simulink library "avlAerodynamics2D"  (R2018b)
settings: Solver=VariableStepAuto  StartTime=0.0  StopTime=10.0  RelTol=1e-3
values from neighbouring files (symbols this model uses):
  Bref = dsgnData.Bref    [avlAerodynamics2D_ts.m]
  Cref = dsgnData.Cref    [avlAerodynamics2D_ts.m]
  k_CS_gain = calculate_2D_gains(dsgnTest_1,nom_a,nom_b,df,da,de,dr)    [avlAero2DCoeffs_ts.m]
  rho_fluid = 1    [avlAerodynamics2D_ts.m]
  Sref = dsgnData.Sref    [avlAerodynamics2D_ts.m]
undefined symbols (not defined in the file or in its folder): CDtot_2D_Tbl, CLtot_2D_Tbl, Cltot_2D_Tbl, Cmtot_2D_Tbl, Cntot_2D_Tbl
libraries: eulAng2RotMat_ul x1, alphaBeta_ul x1, avlAero2DCoeffs_ul x1
settings Model: Creator=mcobb  LastModifiedBy=Ayaz

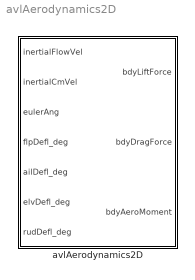
== system avlAerodynamics2D ==
  avlAerodynamics2D : Subsystem  mask{CLTable=CLtot_2D_Tbl, CDTable=CDtot_2D_Tbl, CMxTable=Cltot_2D_Tbl, CMyTable=Cmtot_2D_Tbl, CMzTable=Cntot_2D_Tbl, CsGainMatrix=k_CS_gain, SRef=Sref, BRef=Bref, CRef=Cref, rho_fluid=rho_fluid}
      mask prompts: CLTable "CL lookup table object"; CDTable "CD lookup table object"; CMxTable "CMx lookup table object"; CMyTable "CMy lookup table object"; CMzTable "CMz lookup table object"; CsGainMatrix "Control surface gain matrix"; SRef "Ref area (AVL Sref)"; BRef "Roll & Yaw Moment Reference Length (AVL Bref)"; CRef "Pitch Moment Reference Length (AVL Cref)"; rho_fluid "Fluid density"
      mask TypeOptions CLTable: avlAero2DCoeffs/CLTable
      mask TypeOptions CDTable: avlAero2DCoeffs/CDTable
      mask TypeOptions CMxTable: avlAero2DCoeffs/CMxTable
      mask TypeOptions CMyTable: avlAero2DCoeffs/CMyTable
      mask TypeOptions CMzTable: avlAero2DCoeffs/CMzTable
      mask TypeOptions CsGainMatrix: avlAero2DCoeffs/CsGainMatrix
      mask DialogControl Container4 Prompt: Reference Areas
      mask DialogControl Container5 Prompt: Environment

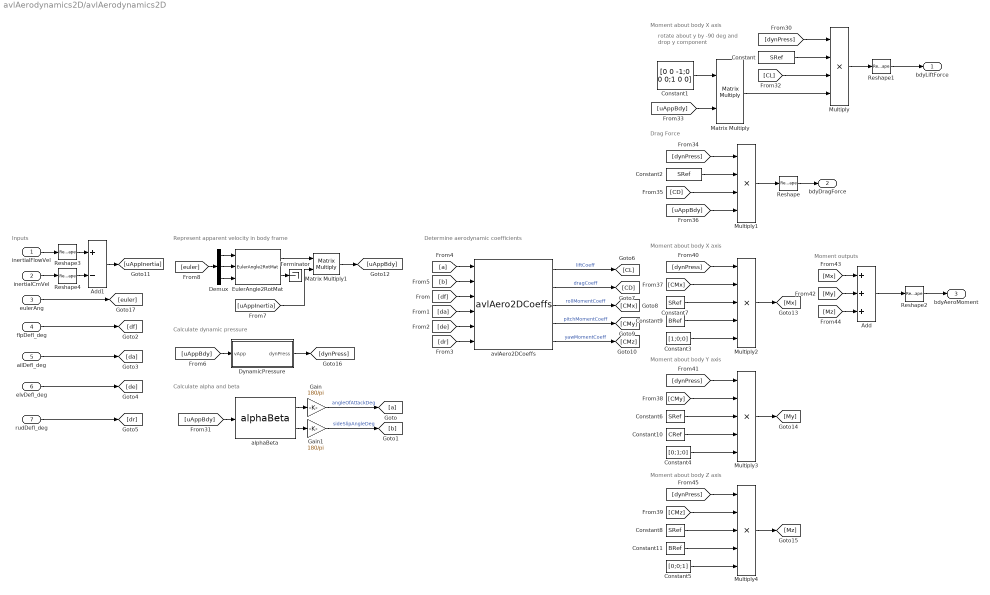
== system avlAerodynamics2D/avlAerodynamics2D ==
  note: Calculate dynamic pressure
  note: Represent apparent velocity in body frame
  note: Moment outputs
  note: Inputs
  note: Calculate alpha and beta
  note: Determine aerodynamic coefficients
  note: Moment about body X axis
  note: rotate about y by -90 deg
      | and drop y component
  note: Moment about body Y axis
  note: Moment about body Z axis
  note: Drag Force
  note: Moment about body X axis
  inertialFlowVel : Inport
  inertialCmVel : Inport  Port=2
  eulerAng : Inport  Port=3
  flpDefl_deg : Inport  Port=4
  ailDefl_deg : Inport  Port=5
  elvDefl_deg : Inport  Port=6
  rudDefl_deg : Inport  Port=7
  Add : Sum  Inputs=+++
  Add1 : Sum  Inputs=+-
  Constant{,2,6..8} (5 alike) : Constant  Value=SRef
  Constant1 : Constant  Value=[0 0 -1;0 0 0;1 0 0]
  Constant10 : Constant  Value=CRef
  Constant11 : Constant  Value=BRef
  Constant3 : Constant  Value=[1;0;0]  VectorParams1D=off
  Constant4 : Constant  Value=[0;1;0]  VectorParams1D=off
  Constant5 : Constant  Value=[0;0;1]  VectorParams1D=off
  Constant9 : Constant  Value=BRef
  Demux : Demux  Outputs=3
  DynamicPressure : Subsystem  mask{rho=rho_fluid}
      mask prompts: rho "Fluid density"
  EulerAngle2RotMat : eulAng2RotMat_ul/EulerAngle2RotMat  SystemSampleTime=-1
  Gain : Gain  Gain=180/pi
  Gain1 : Gain  Gain=180/pi
  Matrix Multiply : Product  Multiplication=Matrix(*)
  Matrix Multiply1 : Product  Multiplication=Matrix(*)
  Multiply : Product  Inputs=4
  Multiply1 : Product  Inputs=4
  Multiply2 : Product  Inputs=5
  Multiply3 : Product  Inputs=5
  Multiply4 : Product  Inputs=5
  Reshape{,1..4} (5 alike) : Reshape  OutputDimensionality=Column vector (2-D)
  Terminator : Terminator
  alphaBeta : alphaBeta_ul/alphaBeta  SystemSampleTime=-1
  avlAero2DCoeffs : avlAero2DCoeffs_ul/avlAero2DCoeffs  CLTable=CLTable  CDTable=CDTable  CMxTable=CMxTable  CMyTable=CMyTable  CMzTable=CMzTable  CsGainMatrix=CsGainMatrix
  bdyLiftForce : Outport
  bdyDragForce : Outport  Port=2
  bdyAeroMoment : Outport  Port=3
  wires:
  flpDefl_deg/1 -> [df]
  ailDefl_deg/1 -> [da]
  elvDefl_deg/1 -> [de]
  rudDefl_deg/1 -> [dr]
  alphaBeta/1 -> Gain/1
  alphaBeta/2 -> Gain1/1
  Gain/1 -> [a]  "angleOfAttackDeg"
  Gain1/1 -> [b]  "sideSlipAngleDeg"
  [uAppBdy] -> alphaBeta/1
  [dynPress] -> Multiply/1
  Constant/1 -> Multiply/2
  [CL] -> Multiply/3
  Matrix Multiply/1 -> Multiply/4
  Constant1/1 -> Matrix Multiply/1
  [uAppBdy] -> Matrix Multiply/2
  [CD] -> Multiply1/3
  Constant2/1 -> Multiply1/2
  [dynPress] -> Multiply1/1
  [uAppBdy] -> Multiply1/4
  Multiply/1 -> Reshape1/1
  Multiply1/1 -> Reshape/1
  Reshape1/1 -> bdyLiftForce/1
  Reshape/1 -> bdyDragForce/1
  [CMx] -> Multiply2/2
  Multiply2/1 -> [Mx]
  Multiply3/1 -> [My]
  [CMy] -> Multiply3/2
  [CMz] -> Multiply4/2
  Multiply4/1 -> [Mz]
  [My] -> Add/2
  [Mx] -> Add/1
  [Mz] -> Add/3
  Add/1 -> Reshape2/1
  Reshape2/1 -> bdyAeroMoment/1
  Reshape3/1 -> Add1/1
  Constant7/1 -> Multiply2/3
  Constant6/1 -> Multiply3/3
  Constant8/1 -> Multiply4/3
  Constant3/1 -> Multiply2/5
  Constant4/1 -> Multiply3/5
  Constant5/1 -> Multiply4/5
  [dynPress] -> Multiply3/1
  [dynPress] -> Multiply4/1
  Constant9/1 -> Multiply2/4
  [dynPress] -> Multiply2/1
  Constant10/1 -> Multiply3/4
  Constant11/1 -> Multiply4/4
  [dr] -> avlAero2DCoeffs/6
  [de] -> avlAero2DCoeffs/5
  [da] -> avlAero2DCoeffs/4
  [df] -> avlAero2DCoeffs/3
  avlAero2DCoeffs/5 -> [CMz]  "yawMomentCoeff"
  avlAero2DCoeffs/4 -> [CMy]  "pitchMomentCoeff"
  avlAero2DCoeffs/3 -> [CMx]  "rollMomentCoeff"
  avlAero2DCoeffs/2 -> [CD]  "dragCoeff"
  avlAero2DCoeffs/1 -> [CL]  "liftCoeff"
  Reshape4/1 -> Add1/2
  eulerAng/1 -> [euler]
  inertialCmVel/1 -> Reshape4/1
  inertialFlowVel/1 -> Reshape3/1
  Add1/1 -> [uAppInertia]
  Demux/1 -> EulerAngle2RotMat/1
  Demux/2 -> EulerAngle2RotMat/2
  Demux/3 -> EulerAngle2RotMat/3
  [euler] -> Demux/1
  EulerAngle2RotMat/2 -> Terminator/1
  EulerAngle2RotMat/1 -> Matrix Multiply1/1
  [uAppInertia] -> Matrix Multiply1/2
  Matrix Multiply1/1 -> [uAppBdy]
  DynamicPressure/1(dynPress) -> [dynPress]
  [uAppBdy] -> DynamicPressure/1(vApp)
  [b] -> avlAero2DCoeffs/2
  [a] -> avlAero2DCoeffs/1

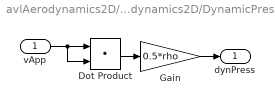
== system avlAerodynamics2D/avlAerodynamics2D/DynamicPressure ==
  vApp : Inport
  Dot Product : DotProduct  InputSameDT=on  OutDataTypeStr=Inherit: Inherit via internal rule
  Gain : Gain  Gain=0.5*rho
  dynPress : Outport
  wires:
  Gain/1 -> dynPress/1
  vApp/1 -> Dot Product/2, Dot Product/1
  Dot Product/1 -> Gain/1
